simulink model "chap8_2sim"  (Simulink 8.1)
settings: Solver=ode45  StartTime=0.0  StopTime=30  RelTol=1e-3
settings Model: Creator=Administrator  LastModifiedBy=liujk
settings DataIOCC: SignalLoggingName=sigsOut
settings OptimizationCC: ExpressionDepthLimit=128  InitFltsAndDblsToZero=on
settings DebuggingCC: SaveWithParameterizedLinksMsg=none  SignalResolutionControl=TryResolveAllWithWarning  SolverPrmCheckMsg=none  MultiTaskDSMMsg=warning  MultiTaskCondExecSysMsg=none  StrictBusMsg=None
settings HardwareCC: TargetUnknown=on
settings RTWCC: IncludeERTFirstTime=on
settings GRTTargetCC: TargetFcnLib=ansi_tfl_tmw.mat

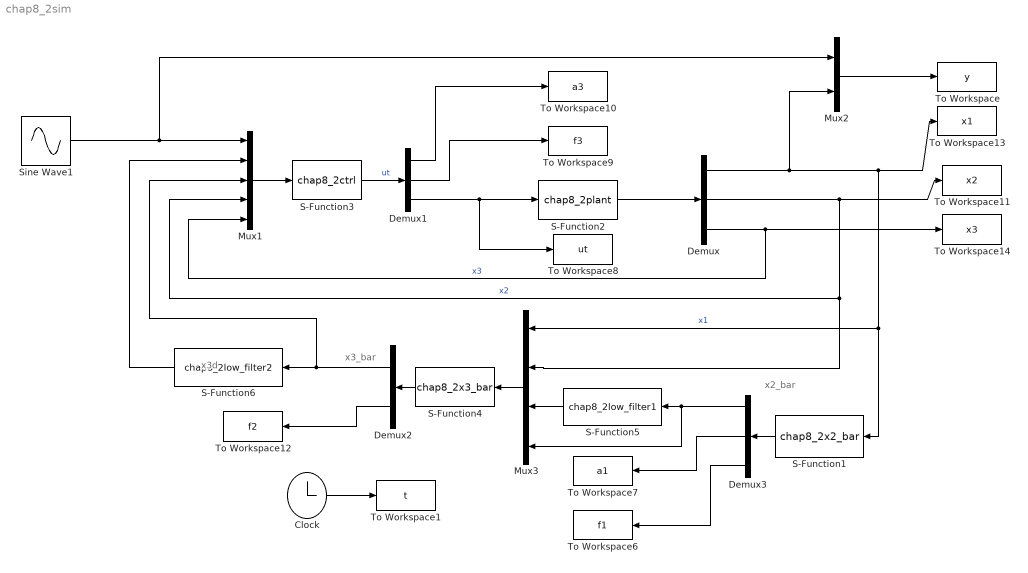
== system chap8_2sim ==
  note: x2_bar
  note: x3_bar
  note: x3d
  Clock : Clock
  Demux : Demux  Outputs=3
  Demux1 : Demux  Outputs=3
  Demux2 : Demux  Outputs=2
  Demux3 : Demux  Outputs=3
  Mux1 : Mux  Inputs=5
  Mux2 : Mux  Inputs=2
  Mux3 : Mux
  S-Function1 : S-Function  FunctionName=chap8_2x2_bar  EnableBusSupport=off
  S-Function2 : S-Function  FunctionName=chap8_2plant  EnableBusSupport=off
  S-Function3 : S-Function  FunctionName=chap8_2ctrl  EnableBusSupport=off
  S-Function4 : S-Function  FunctionName=chap8_2x3_bar  EnableBusSupport=off
  S-Function5 : S-Function  FunctionName=chap8_2low_filter1  EnableBusSupport=off
  S-Function6 : S-Function  FunctionName=chap8_2low_filter2  EnableBusSupport=off
  Sine Wave1 : Sin  Amplitude=5  SampleTime=0
  To Workspace : ToWorkspace  VariableName=y  SampleTime=-1
  To Workspace1 : ToWorkspace  VariableName=t  SampleTime=-1
  To Workspace10 : ToWorkspace  VariableName=a3  SampleTime=-1
  To Workspace11 : ToWorkspace  VariableName=x2  SampleTime=-1
  To Workspace12 : ToWorkspace  VariableName=f2  SampleTime=-1
  To Workspace13 : ToWorkspace  VariableName=x1  SampleTime=-1
  To Workspace14 : ToWorkspace  VariableName=x3  SampleTime=-1
  To Workspace6 : ToWorkspace  VariableName=f1  SampleTime=-1
  To Workspace7 : ToWorkspace  VariableName=a1  SampleTime=-1
  To Workspace8 : ToWorkspace  VariableName=ut  SampleTime=-1
  To Workspace9 : ToWorkspace  VariableName=f3  SampleTime=-1
  wires:
  Clock/1 -> To Workspace1/1
  Mux1/1 -> S-Function3/1
  Sine Wave1/1 -> Mux2/1, Mux1/1
  S-Function2/1 -> Demux/1
  Demux/1 -> Mux2/2, Mux3/1, S-Function1/1, To Workspace13/1  "x1"
  Mux2/1 -> To Workspace/1
  Mux3/1 -> S-Function4/1
  Demux/3 -> To Workspace14/1, Mux1/5  "x3"
  S-Function6/1 -> Mux1/2
  S-Function5/1 -> Mux3/3
  Demux/2 -> Mux3/2, Mux1/4, To Workspace11/1  "x2"
  S-Function3/1 -> Demux1/1  "ut"
  Demux1/3 -> S-Function2/1, To Workspace8/1
  Demux1/1 -> To Workspace10/1
  Demux1/2 -> To Workspace9/1
  S-Function4/1 -> Demux2/1
  Demux2/1 -> S-Function6/1, Mux1/3
  Demux2/2 -> To Workspace12/1
  S-Function1/1 -> Demux3/1
  Demux3/1 -> S-Function5/1, Mux3/4
  Demux3/3 -> To Workspace6/1
  Demux3/2 -> To Workspace7/1
